simulink model "mpptproject_IncCon_MPPT"  (R2026a)
settings: Solver=FixedStepAuto  StopTime=200
model workspace (MAT data in the model file):
  deltaD = 0.01
undefined symbols (not defined in the file): epsilone, epsilonI, epsilonV
libraries: nesl_utility x5, simulink x5, fl_lib x4, ee_lib x2
settings Model: Creator=jacks  LastModifiedBy=jacks

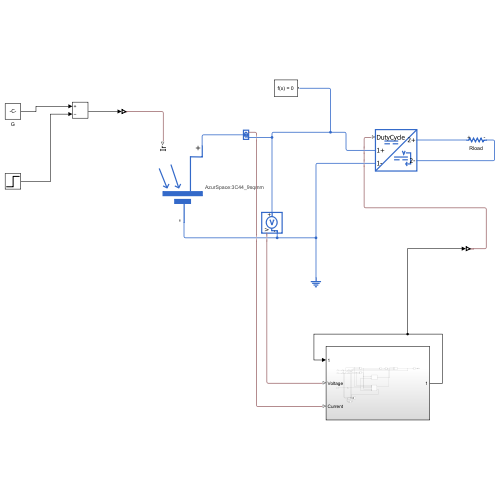
[thumbnail: Simulink's stored preview of the top-level diagram]
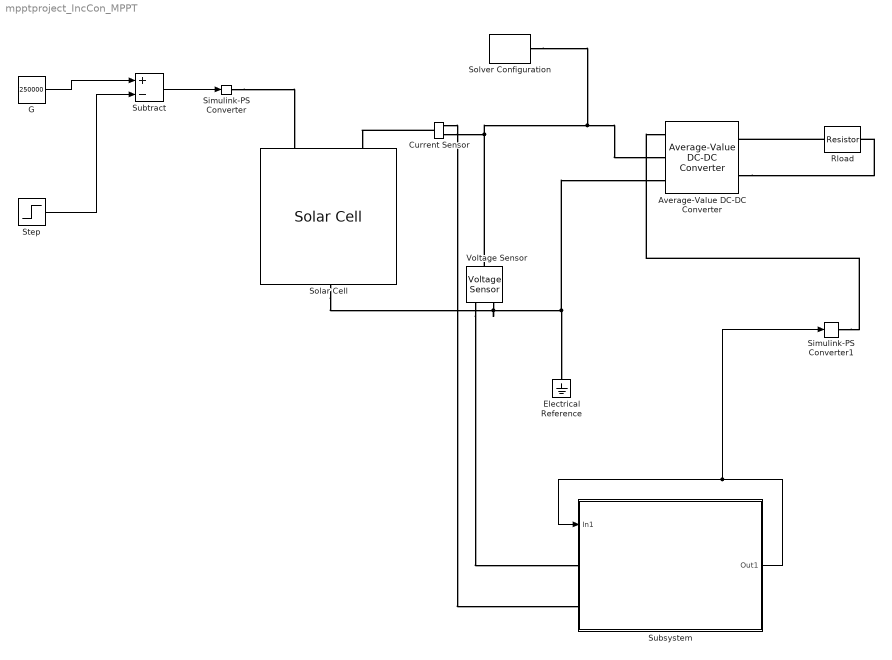
== system mpptproject_IncCon_MPPT ==
  Average-Value DC-DC Converter : ee_lib/Semiconductors & Converters/Converters/Average-Value DC-DC Converter  implementation_option=ee.enum.converters.implementation.averageValue  converter_type=ee.enum.converters.dcdctype.boost  control_option=ee.enum.converters.controlinput.dutycycle  efficiency_option=ee.enum.converters.efficiency.constant  efficiency_fixed=100  i_vec=[0, 2, 5] A  efficiency_vec=[90, 95, 98]  Lf=100e-6 H  Rl=0 Ohm  Cf=100e-6 F  Rc=1e-6 Ohm  iL_specify=off  iL_priority=High  iL=0 A  iL_nominal_specify=off  iL_nominal_value=1  iL_nominal_unit=A  vc_specify=off  vc_priority=High  vc=0 V  vc_nominal_specify=off  vc_nominal_value=1  vc_nominal_unit=V
  Current Sensor : fl_lib/Electrical/Electrical Sensors/Current Sensor
  Electrical Reference : fl_lib/Electrical/Electrical Elements/Electrical Reference
  G : Constant  Value=250000
  Rload : fl_lib/Electrical/Electrical Elements/Resistor  R=25 Ohm  i_specify=off  i_priority=None  i=0 A  i_nominal_specify=off  i_nominal_value=1  i_nominal_unit=A  v_specify=off  v_priority=None  v=0 V  v_nominal_specify=off  v_nominal_value=1  v_nominal_unit=V
  Simulink-PS Converter : nesl_utility/Simulink-PS Converter  PhysicalDomain=network_engine_domain  SubClassName=ps_input  LeftPortType=input  RightPortType=output  PseudoPeriodic=off  Frequencies=[]  NoiseDistribution=none  NoiseParameters=[]  Unit=1  AffineConversion=off  FilteringAndDerivatives=provide  SimscapeFilterOrder=1  InputFilterTimeConstant=0.001  UdotUserProvided=0
  Simulink-PS Converter1 : nesl_utility/Simulink-PS Converter  PhysicalDomain=network_engine_domain  SubClassName=ps_input  LeftPortType=input  RightPortType=output  PseudoPeriodic=off  Frequencies=[]  NoiseDistribution=none  NoiseParameters=[]  Unit=1  AffineConversion=off  FilteringAndDerivatives=provide  SimscapeFilterOrder=1  InputFilterTimeConstant=0.001  UdotUserProvided=0
  Solar Cell : ee_lib/Sources/Solar Cell  PartSpecification="{\"CollectionId\":\"MW.SimscapeElectrical\",\"CollectionVersion\":\"1.0.0\",\"DatasetId\":\"AzurSpace|3C44_9sqmm|simscape.electrical.solarCell\",\"DisplayName\":\"AzurSpace:3C44_9sqmm\"}"  prm=ee.enum.sources.solar_cell_prm.eightParameter  Isc=0.37 % Datasheet derived A  Voc=3.05 % Datasheet derived V  Is=1.91003784590348e-35 % Datasheet derived A  Is2=8.42205890783812e-38 % Datasheet derived A  Iph=0.370001258541474 % Datasheet derived A  Ir0=250000 % Datasheet derived W/m^2  ec=1.50364371134548 % Datasheet derived  N2=1.73316940278898 % Datasheet derived  Rs=0.306625056084457 % Datasheet derived Ohm  Rp=90147.3159723304 % Datasheet derived Ohm  N_series=1 % Datasheet derived  N_parallel=1 % Datasheet derived  TIPH1=0.000800010328673928 % Datasheet derived 1/K  EG=1.441 % Datasheet derived eV  TXIS1=104.115941100637 % Datasheet derived  TXIS2=5.57230100941371 % Datasheet derived  TRS1=0.775797800706674 % Datasheet derived  TRP1=0 % Parameter not set  Tmeas=25 % Datasheet derived degC  TFIXED=25 % Datasheet derived degC  thermal_mass=100 % Parameter not set J/K  initial_temperature=25 degC
      settings: AttributesFormatString=AzurSpace:3C44_9sqmm
  Solver Configuration : nesl_utility/Solver Configuration  PhysicalDomain=network_engine_domain  SubClassName=solver  LeftPortType=input  RightPortType=generic  Tones=[]  Harmonics=[]  SimulateNoise=off  Profile=off  UseLocalSampling=off  EnableSwitchedLinearOptims=on  FrequencyDomain=off  UseCCode=off  RelTol=0.001  AbsTol=0.001  MinStep=1e-09  ToWorkspace=off  RevertToSquareIcSolve=off  NumHomotopyIterations=100  PhasorMode=off  PhasorModeNumHarmonics=1  ConsistencySolver=NEWTON_XTOL_AFTER_FTOL  CanonicalOrdering=CANONICAL  OptimizeIntermediates=OPTIMIZED  IndexReductionMethod=DerivativeReplacement  DoDC=off  ResidualTolerance=1e-09  ConsistencyTolSource=GLOBAL  ConsistencyAbsTol=0.001  ConsistencyRelTol=0.001  ConsistencyTolFactor=0.001  UseLocalSolver=off  LocalSolverChoice=NE_BACKWARD_EULER_ADVANCER  ResolveIndetEquations=on  FunctionEvalNumThread=1  LocalSolverSampleTime=0.001  DoFixedCost=off  MaxNonlinIter=3  MaxModeIter=2  ComputeImpulses=off  ImpulseIterations=2  LinearAlgebra=auto  LinearAlgebraNumThread=0  EquationFormulation=NE_TIME_EF  DelaysMemoryBudget=1024  AutomaticFiltering=on  FilteringTimeConstant=0.001  PartitionStorageMethod=AS_NEEDED  PartitionMemoryBudget=1024  PartitionMethod=ROBUST  MultibodyUseLocalSolver=off  MultibodyLocalSolverChoice=ODE1  MultibodyLocalSolverSampleTime=0.001
  Step : Step  Time=100  FinalValue=100000  SampleTime=0
  Subsystem : Subsystem
  Subtract : Sum  Inputs=+-
  Voltage Sensor : fl_lib/Electrical/Electrical Sensors/Voltage Sensor
  wires:
  Subsystem/1(Out1) -> Simulink-PS Converter1/1, Subsystem/1(In1)
  Step/1 -> Subtract/2
  G/1 -> Subtract/1
  Subtract/1 -> Simulink-PS Converter/1
  connections:
  Simulink-PS Converter/RConn1 -- Solar Cell/LConn1
  Voltage Sensor/LConn1 -- Solver Configuration/RConn1 -- Average-Value DC-DC Converter/LConn2 -- Current Sensor/RConn2
  Solar Cell/RConn1 -- Voltage Sensor/RConn2 -- Average-Value DC-DC Converter/LConn3 -- Electrical Reference/LConn1
  Rload/LConn1 -- Average-Value DC-DC Converter/RConn1
  Average-Value DC-DC Converter/RConn2 -- Rload/RConn1
  Voltage Sensor/RConn1 -- Subsystem/LConn1
  Current Sensor/LConn1 -- Solar Cell/LConn2
  Current Sensor/RConn1 -- Subsystem/LConn2
  Simulink-PS Converter1/RConn1 -- Average-Value DC-DC Converter/LConn1

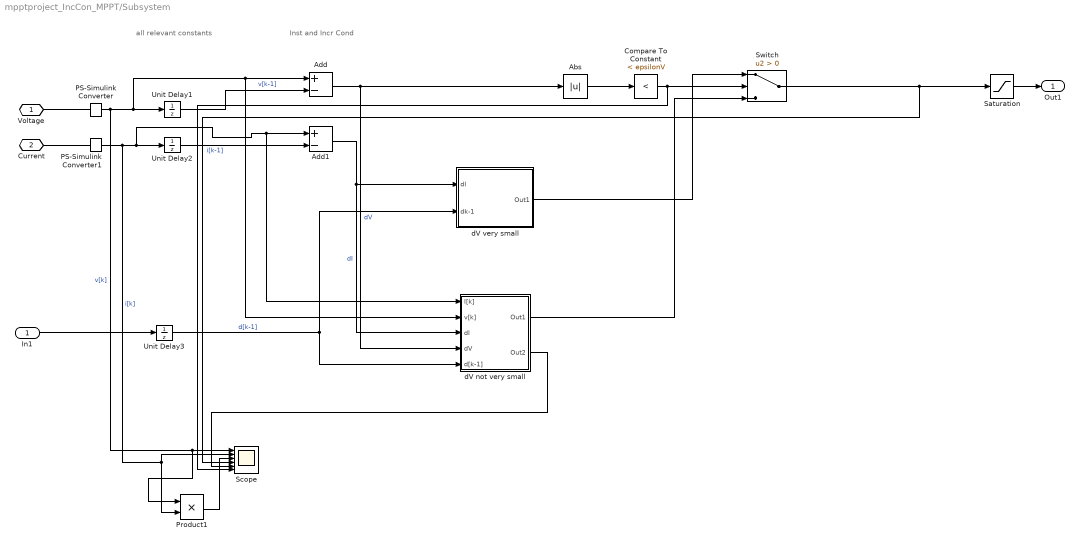
== system mpptproject_IncCon_MPPT/Subsystem ==
  note: Inst and Incr Cond
  note: all relevant constants
  In1 : Inport
  Abs : Abs  SaturateOnIntegerOverflow=off
  Add : Sum  Inputs=+-
  Add1 : Sum  Inputs=+-
  Compare To Constant : simulink/Logic and Bit Operations/Compare To Constant  relop=<  const=epsilonV  OutDataTypeStr=boolean
  PS-Simulink Converter : nesl_utility/PS-Simulink Converter  PhysicalDomain=network_engine_domain  SubClassName=ps_output  LeftPortType=input  RightPortType=output  PseudoPeriodic=off  Frequencies=[]  VectorFormat=inherit  Unit=inherit  AffineConversion=off
  PS-Simulink Converter1 : nesl_utility/PS-Simulink Converter  PhysicalDomain=network_engine_domain  SubClassName=ps_output  LeftPortType=input  RightPortType=output  PseudoPeriodic=off  Frequencies=[]  VectorFormat=inherit  Unit=inherit  AffineConversion=off
  Product1 : Product
  Saturation : Saturate  UpperLimit=0.8  LowerLimit=0.05
  Scope : Scope  NumInputPorts=6
      settings: ActiveDisplayYMinimum=-3.330739603870986  ActiveDisplayYMaximum=4.3920097895003618
  Switch : Switch  Criteria=u2 > Threshold  SaturateOnIntegerOverflow=off  InputSameDT=off
  Unit Delay1 : UnitDelay  InitialCondition=1  SampleTime=-1
  Unit Delay2 : UnitDelay  InitialCondition=1  SampleTime=-1
  Unit Delay3 : UnitDelay  InitialCondition=1  SampleTime=-1
  dV not very small : Subsystem
  dV very small : Subsystem
  Voltage : PMIOPort  Side=Left
  Current : PMIOPort  Port=2  Side=Left
  Out1 : Outport
  wires:
  PS-Simulink Converter/1 -> Product1/1, Scope/1, dV not very small/2(v[k]), Add/1, Unit Delay1/1  "v[k]"
  PS-Simulink Converter1/1 -> Scope/2, Product1/2, dV not very small/1(I[k]), Add1/1, Unit Delay2/1  "i[k]"
  Unit Delay2/1 -> Add1/2  "i[k-1]"
  Unit Delay1/1 -> Add/2  "v[k-1]"
  In1/1 -> Unit Delay3/1
  Product1/1 -> Scope/3
  Abs/1 -> Compare To Constant/1
  Add/1 -> dV not very small/4(dV), Abs/1  "dV"
  Compare To Constant/1 -> Scope/6, Switch/2
  Add1/1 -> dV not very small/3(dI), dV very small/1(dI)  "dI"
  Unit Delay3/1 -> dV very small/2(dk-1), dV not very small/5(d[k-1])  "d[k-1]"
  dV very small/1(Out1) -> Switch/1
  dV not very small/1(Out1) -> Switch/3
  Switch/1 -> Saturation/1, Scope/4
  Saturation/1 -> Out1/1
  dV not very small/2(Out2) -> Scope/5
  connections:
  Voltage/RConn1 -- PS-Simulink Converter/LConn1
  Current/RConn1 -- PS-Simulink Converter1/LConn1

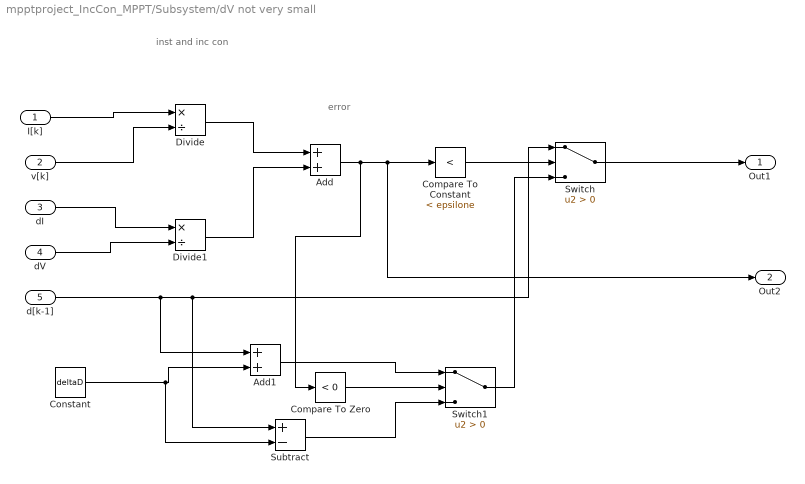
== system mpptproject_IncCon_MPPT/Subsystem/dV not very small ==
  note: error
  note: inst and inc con
  I[k] : Inport
  v[k] : Inport  Port=2
  dI : Inport  Port=3
  dV : Inport  Port=4
  d[k-1] : Inport  Port=5
  Add : Sum
  Add1 : Sum
  Compare To Constant : simulink/Logic and Bit Operations/Compare To Constant  relop=<  const=epsilone  OutDataTypeStr=boolean
  Compare To Zero : simulink/Logic and Bit Operations/Compare To Zero  relop=<  OutDataTypeStr=boolean
  Constant : Constant  Value=deltaD
  Divide : Product  Inputs=*/
  Divide1 : Product  Inputs=*/
  Subtract : Sum  Inputs=+-
  Switch : Switch  Criteria=u2 > Threshold  SaturateOnIntegerOverflow=off  InputSameDT=off
  Switch1 : Switch  Criteria=u2 > Threshold  SaturateOnIntegerOverflow=off  InputSameDT=off
  Out1 : Outport
  Out2 : Outport  Port=2
  wires:
  I[k]/1 -> Divide/1
  v[k]/1 -> Divide/2
  dI/1 -> Divide1/1
  dV/1 -> Divide1/2
  Divide/1 -> Add/1
  Divide1/1 -> Add/2
  Compare To Constant/1 -> Switch/2
  Constant/1 -> Subtract/2, Add1/2
  d[k-1]/1 -> Add1/1, Subtract/1, Switch/1
  Switch/1 -> Out1/1
  Add/1 -> Compare To Zero/1, Out2/1, Compare To Constant/1
  Compare To Zero/1 -> Switch1/2
  Add1/1 -> Switch1/1
  Subtract/1 -> Switch1/3
  Switch1/1 -> Switch/3

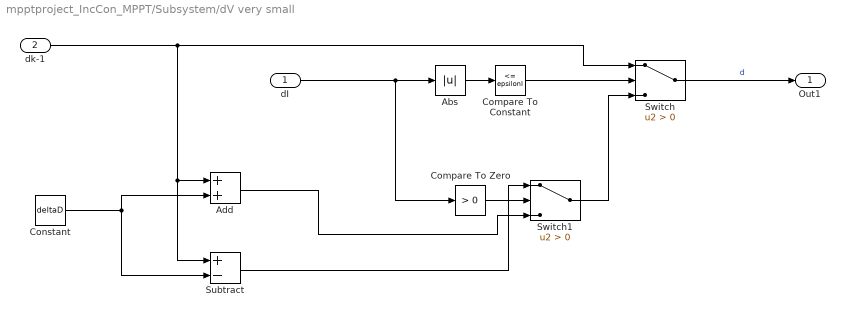
== system mpptproject_IncCon_MPPT/Subsystem/dV very small ==
  dI : Inport
  dk-1 : Inport  Port=2
  Abs : Abs  SaturateOnIntegerOverflow=off
  Add : Sum
  Compare To Constant : simulink/Logic and Bit Operations/Compare To Constant  relop=<=  const=epsilonI  OutDataTypeStr=boolean
  Compare To Zero : simulink/Logic and Bit Operations/Compare To Zero  relop=>  OutDataTypeStr=boolean
  Constant : Constant  Value=deltaD
  Subtract : Sum  Inputs=+-
  Switch : Switch  Criteria=u2 > Threshold  SaturateOnIntegerOverflow=off  InputSameDT=off
  Switch1 : Switch  Criteria=u2 > Threshold  SaturateOnIntegerOverflow=off  InputSameDT=off
  Out1 : Outport
  wires:
  dI/1 -> Compare To Zero/1, Abs/1
  Abs/1 -> Compare To Constant/1
  Compare To Constant/1 -> Switch/2
  Switch/1 -> Out1/1  "d"
  dk-1/1 -> Subtract/1, Add/1, Switch/1
  Compare To Zero/1 -> Switch1/2
  Constant/1 -> Subtract/2, Add/2
  Switch1/1 -> Switch/3
  Subtract/1 -> Switch1/1
  Add/1 -> Switch1/3
